simulink model "ArduCopter_MinnieTrajController"  (R2018b)
settings: Solver=FixedStepDiscrete  StartTime=0.0  StopTime=1000  FixedStep=cntrl.sample_time  RelTol=1e-4
undefined symbols (not defined in the file): cycle, DiscIntNeverNeededParam, fm_loiter, traj_empty
libraries: simulink x6, ndi_lib x5, axes_transformation_lib x4, angles_lib x3, ardupilot_custom_controller_lib x2, filters_lib x2, cntrl_atti_red_indi_lib x2, traj_lib x2, control_allocation_lib x1, dspsigops x1
(part 1 of 2)
settings Model: Creator=Yannic  LastModifiedBy=eike
settings SolverCC: ZeroCrossControl=DisableAll
settings DataIOCC: LimitDataPoints=on  SaveOutput=off  SaveTime=off  ReturnWorkspaceOutputs=on
settings OptimizationCC: DefaultParameterBehavior=Inlined  UseFloatMulNetSlope=on  DefaultUnderspecifiedDataType=single  InlineInvariantSignals=on  PassReuseOutputArgsAs=Individual arguments  ZeroExternalMemoryAtStartup=off  ZeroInternalMemoryAtStartup=off  NoFixptDivByZeroProtection=on  EfficientFloat2IntCast=on  LifeSpan=1  OptimizeBlockOrder=speed  DifferentSizesBufferReuse=on
settings DebuggingCC: ReadBeforeWriteMsg=DisableAll  WriteAfterWriteMsg=DisableAll  WriteAfterReadMsg=DisableAll  MultiTaskDSMMsg=none  ParameterTunabilityLossMsg=error  AllowSymbolicDim=off  LibraryContextMissingDiagnostic=none  SFUnexpectedBacktrackingDiag=warning  SFNoUnconditionalDefaultTransitionDiag=warning  SFExecutionAtInitializationDiag=none
settings HardwareCC: ProdBitPerPointer=32  ProdBitPerSizeT=32  ProdBitPerPtrDiffT=32  ProdLargestAtomicInteger=Long  ProdLargestAtomicFloat=Double  ProdWordSize=32  ProdHWDeviceType=ARM Compatible->ARM Cortex
settings ModelReferenceCC: UpdateModelReferenceTargets=IfOutOfDate  PropagateSignalLabelsOutOfModel=off
settings SFSimCC: SFSimEcho=off  SimUseLocalCustomCode=off  MATLABDynamicMemAlloc=off
settings RTWCC: SystemTargetFile=ert.tlc  GenCodeOnly=on  TemplateMakefile=ert_default_tmf  GenerateReport=on  RTWUseLocalCustomCode=off  IncludeHyperlinkInReport=on  LaunchReport=on  TargetLang=C++  GenerateTraceInfo=on  GenerateTraceReport=on  GenerateTraceReportSl=on  GenerateTraceReportSf=on  GenerateTraceReportEml=on
settings CodeAppCC: ForceParamTrailComments=on  IgnoreCustomStorageClasses=off  OperatorAnnotations=on  SimulinkDataObjDesc=on  SFDataObjDesc=on  CustomSymbolStrGlobalVar=rt$N$M  CustomSymbolStrType=$N$M  CustomSymbolStrFcn=$N$M$F  CustomSymbolStrMacro=$N$M  InsertBlockDesc=on
settings ERTTargetCC: TargetLangStandard=C++03 (ISO)  GenerateSampleERTMain=on  IncludeMdlTerminateFcn=off  CombineSignalStateStructs=on  SuppressErrorStatus=on  SupportAbsoluteTime=off  MultiInstanceERTCode=on  CodeInterfacePackaging=C++ class  SupportVariableSizeSignals=on  ERTHeaderFileRootName=MatlabController$E  ERTSourceFileRootName=MatlabController$E  ERTDataFileRootName=MatlabController_data  InlinedParameterPlacement=NonHierarchical  RootIOFormat=Structure reference  ERTCustomFileTemplate=example_file_process.tlc  ERTFilePackagingFormat=CompactWithDataFile
settings ConfigComp: CovMetricSettings=dw  CovHtmlReporting=on  CovSaveCumulativeToWorkspaceVar=on  CovSaveSingleToWorkspaceVar=on  CovExternalEMLEnable=off

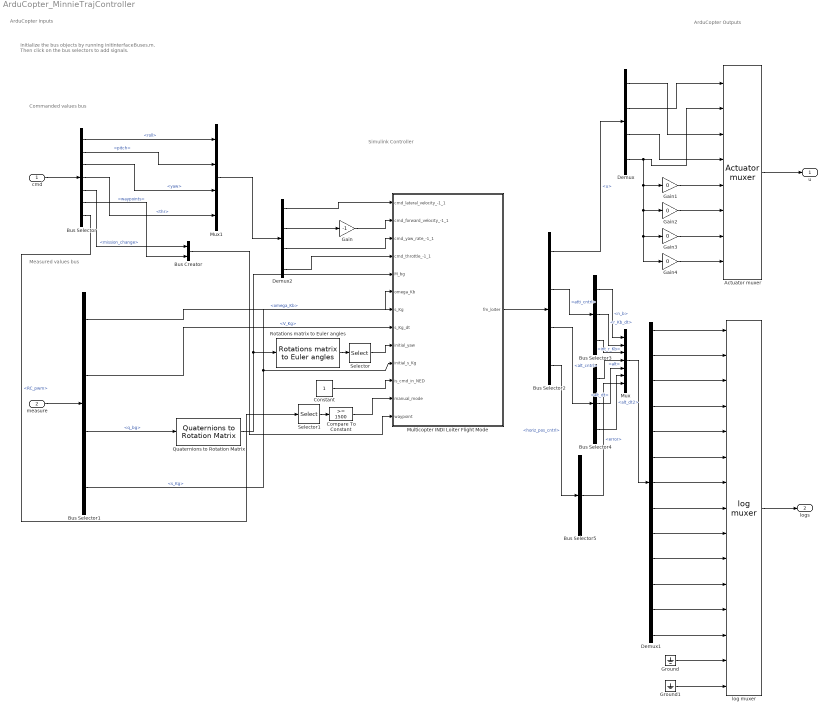
== system ArduCopter_MinnieTrajController ==
  note: Measured values bus
  note: Initialize the bus objects by running initInterfaceBuses.m.
      | Then click on the bus selectors to add signals.
  note: Commanded values bus
  note: ArduCopter Inputs
  note: ArduCopter Outputs
  note: Simulink Controller
  cmd : Inport  OutDataTypeStr=Bus: cmdBus
  measure : Inport  Port=2  OutDataTypeStr=Bus: measureBus
  Actuator muxer : ardupilot_custom_controller_lib/Actuator muxer
      settings: SourceProductName=LADAC
  Bus Creator : BusCreator  Inputs=2
  Bus Selector : BusSelector  OutputSignals=roll,pitch,yaw,thr,mission_change,waypoints,RC_pwm
  Bus Selector1 : BusSelector  OutputSignals=omega_Kb,V_Kg,q_bg,s_Kg
  Bus Selector2 : BusSelector  OutputSignals=fm_alt_hold.u,fm_alt_hold.atti_cntrl,fm_alt_hold.alt_cntrl,horiz_pos_cntrl
  Bus Selector3 : BusSelector  OutputSignals=error.n_b,error.r_Kb_dt,error.int_r_Kb
  Bus Selector4 : BusSelector  OutputSignals=error.alt,error.alt_dt,error.alt_dt2
  Bus Selector5 : BusSelector  OutputSignals=error
  Compare To Constant : simulink/Logic and Bit Operations/Compare To Constant  relop=>=  const=1500  OutDataTypeStr=boolean
  Constant : Constant
  Demux : Demux
  Demux1 : Demux  Outputs=13
  Demux2 : Demux
  Gain : Gain  Gain=-1
  Gain{1..4} (4 alike) : Gain  Gain=0
  Ground : Ground
  Ground1 : Ground
  Multicopter INDI Loiter Flight Mode : Subsystem  AncestorBlock=fm_copter_loiter_indi_lib/Multicopter INDI Loiter Flight Mode  mask{fm=fm_loiter}
      mask prompts: fm "Multicopter INDI loiter flight  struct"
      mask DialogControl DescGroupVar Prompt: Multicopter INDI Loiter Flight Mode
      mask DialogControl DescTextVar Prompt: Loiter flight mode using the reduced attitude controller with INDI.
      mask DialogControl Control2 Prompt: To intialize the parameters struct see multicopterFlightModeLoiter.
  Mux : Mux  Inputs=7
  Mux1 : Mux
  Quaternions to Rotation Matrix : axes_transformation_lib/Quaternions to Rotation Matrix  SystemSampleTime=-1
      settings: SourceProductName=LADAC
  Rotations matrix to Euler angles : axes_transformation_lib/Rotations matrix to Euler angles  SystemSampleTime=-1
      settings: SourceProductName=LADAC
  Selector : Selector  InputPortWidth=3  IndexOptions=Index vector (dialog)  Indices=3  OutputSizes=1
  Selector1 : Selector  InputPortWidth=16  IndexOptions=Index vector (dialog)  Indices=7  OutputSizes=1
  log muxer : ardupilot_custom_controller_lib/log muxer
      settings: SourceProductName=LADAC
  u : Outport  OutDataTypeStr=single
  logs : Outport  Port=2  OutDataTypeStr=single
  wires:
  cmd/1 -> Bus Selector/1
  measure/1 -> Bus Selector1/1
  Bus Selector/1 -> Mux1/1  "<roll>"
  Bus Selector/2 -> Mux1/2  "<pitch>"
  Bus Selector/3 -> Mux1/3  "<yaw>"
  Bus Selector/4 -> Mux1/4  "<thr>"
  Actuator muxer/1 -> u/1
  log muxer/1 -> logs/1
  Demux/4 -> Actuator muxer/2, Gain1/1, Gain4/1, Gain3/1, Gain2/1
  Gain1/1 -> Actuator muxer/5
  Demux/3 -> Actuator muxer/4
  Demux/2 -> Actuator muxer/1
  Demux1/1 -> log muxer/1
  Demux1/2 -> log muxer/2
  Demux1/3 -> log muxer/3
  Demux1/4 -> log muxer/4
  Demux1/5 -> log muxer/5
  Demux1/6 -> log muxer/6
  Demux1/7 -> log muxer/7
  Demux1/8 -> log muxer/8
  Demux1/9 -> log muxer/9
  Demux1/10 -> log muxer/10
  Demux1/11 -> log muxer/11
  Demux1/12 -> log muxer/12
  Demux1/13 -> log muxer/13
  Ground/1 -> log muxer/14
  Ground1/1 -> log muxer/15
  Gain/1 -> Multicopter INDI Loiter Flight Mode/2(cmd_forward_velocity_-1_1)
  Quaternions to Rotation Matrix/1 -> Multicopter INDI Loiter Flight Mode/5(M_bg), Rotations matrix to Euler angles/1
  Bus Selector1/2 -> Multicopter INDI Loiter Flight Mode/8(s_Kg_dt)  "<V_Kg>"
  Rotations matrix to Euler angles/1 -> Selector/1
  Mux1/1 -> Demux2/1
  Bus Selector1/1 -> Multicopter INDI Loiter Flight Mode/6(omega_Kb)  "<omega_Kb>"
  Demux2/2 -> Gain/1
  Demux2/3 -> Multicopter INDI Loiter Flight Mode/3(cmd_yaw_rate_-1_1)
  Bus Selector1/4 -> Multicopter INDI Loiter Flight Mode/10(initial_s_Kg), Multicopter INDI Loiter Flight Mode/7(s_Kg)  "<s_Kg>"
  Constant/1 -> Multicopter INDI Loiter Flight Mode/11(is_cmd_in_NED)
  Demux2/1 -> Multicopter INDI Loiter Flight Mode/1(cmd_lateral_velocity_-1_1)
  Bus Selector1/3 -> Quaternions to Rotation Matrix/1  "<q_bg>"
  Multicopter INDI Loiter Flight Mode/1(fm_loiter) -> Bus Selector2/1
  Bus Selector2/1 -> Demux/1  "<u>"
  Gain2/1 -> Actuator muxer/6
  Gain3/1 -> Actuator muxer/7
  Gain4/1 -> Actuator muxer/8
  Demux/1 -> Actuator muxer/3
  Bus Selector2/2 -> Bus Selector3/1  "<atti_cntrl>"
  Bus Selector2/3 -> Bus Selector4/1  "<alt_cntrl>"
  Bus Selector2/4 -> Bus Selector5/1  "<horiz_pos_cntrl>"
  Bus Selector5/1 -> Mux/7  "<error>"
  Bus Selector3/1 -> Mux/1  "<n_b>"
  Bus Selector3/3 -> Mux/3  "<int_r_Kb>"
  Bus Selector4/1 -> Mux/4  "<alt>"
  Bus Selector4/3 -> Mux/6  "<alt_dt2>"
  Mux/1 -> Demux1/1
  Bus Selector4/2 -> Mux/5  "<alt_dt>"
  Bus Selector3/2 -> Mux/2  "<r_Kb_dt>"
  Selector/1 -> Multicopter INDI Loiter Flight Mode/9(initial_yaw)
  Bus Selector/5 -> Bus Creator/1  "<mission_change>"
  Bus Selector/6 -> Bus Creator/2  "<waypoints>"
  Bus Selector/7 -> Selector1/1  "<RC_pwm>"
  Selector1/1 -> Compare To Constant/1
  Compare To Constant/1 -> Multicopter INDI Loiter Flight Mode/12(manual_mode)
  Bus Creator/1 -> Multicopter INDI Loiter Flight Mode/13(waypoint)
  Demux2/4 -> Multicopter INDI Loiter Flight Mode/4(cmd_throttle_-1_1)

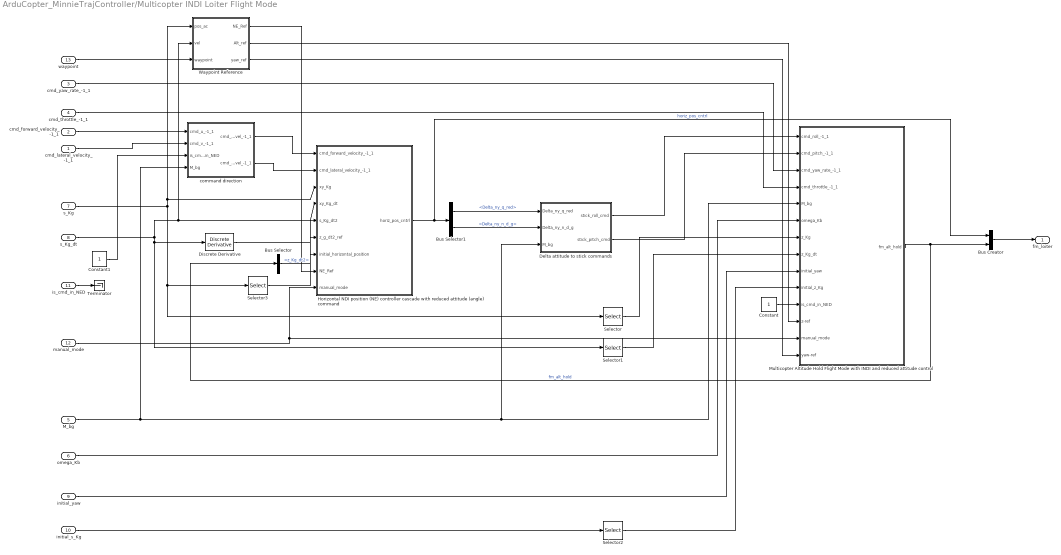
== system ArduCopter_MinnieTrajController/Multicopter INDI Loiter Flight Mode ==
  cmd_lateral_velocity_-1_1 : Inport  SampleTime=fm.sample_time
  cmd_forward_velocity_-1_1 : Inport  Port=2  SampleTime=fm.sample_time
  cmd_yaw_rate_-1_1 : Inport  Port=3  SampleTime=fm.sample_time
  cmd_throttle_-1_1 : Inport  Port=4  SampleTime=fm.sample_time
  M_bg : Inport  Port=5  SampleTime=fm.sample_time
  omega_Kb : Inport  Port=6  SampleTime=fm.sample_time
  s_Kg : Inport  Port=7  SampleTime=fm.sample_time
  s_Kg_dt : Inport  Port=8  SampleTime=fm.sample_time
  initial_yaw : Inport  Port=9  SampleTime=fm.sample_time
  initial_s_Kg : Inport  Port=10  SampleTime=fm.sample_time
  is_cmd_in_NED : Inport  Port=11  SampleTime=fm.sample_time
  manual_mode : Inport  Port=12
  waypoint : Inport  Port=13
  Bus Creator : BusCreator  Inputs=2
  Bus Selector : BusSelector  OutputSignals=alt_cntrl.reference.z_Kg_dt2
  Bus Selector1 : BusSelector  OutputSignals=pseudo_control.Delta_ny_q_red,pseudo_control.Delta_ny_n_d_g
  Constant : Constant
  Constant1 : Constant  OutDataTypeStr=Inherit: Inherit via back propagation
  Delta attitude to stick commands : Subsystem
  Discrete Derivative : simulink/Discrete/Discrete Derivative  gainval=1.0  ICPrevScaledInput=0.0  OutMin=[]  OutMax=[]  OutDataType=fixdt(1, 16)  OutScaling=2^-10  DoSatur=off
  Horizontal NDI position (NE) controller cascade with reduced attitude (angle) command : Subsystem  AncestorBlock=|  mask{horiz_pos_cntrl=fm.horiz_pos_cntrl, T=2./fm.fm_alt.cntrl.atti_cntrl.rm.lean.omega + fm.fm_alt.motor_time_constant + 2./fm.fm_alt.sens_filt.omega}
      | cntrl_horiz_pos_indi_lib/Horizontal NDI position (NE) controller cascade
      | with reduced attitude (angle) command
      mask prompts: horiz_pos_cntrl "horizontal position controller struct"; T "inner loop time constant"
      mask DialogControl DescGroupVar Prompt: Horizontal position controller cascade
      mask DialogControl DescTextVar Prompt: The commanded velocity is filtered and the control error is converted into desired accerlations in x_g and y_g direction. The commanded accelerations are converted into commanded to reduced attitude angles.
      mask DialogControl Control2 Prompt: To initialize a horizontal position controller parameters struct see cntrlHorizPosIndiLoadParams
  Multicopter Altitude Hold Flight Mode with INDI and reduced attitude control : Subsystem  AncestorBlock=fm_copter_alt_hold_indi_lib/Multicopter Altitude Hold Flight Mode with INDI and reduced attitude control  mask{fm=fm.fm_alt}
      mask prompts: fm "Multicopter Altitude Hold Flight Mode (INDI) struct"
      mask DialogControl DescGroupVar Prompt: Multicopter Attitude Flight Mode with INDI and reduced attitude control
      mask DialogControl DescTextVar Prompt: Controller is basically implemented according to [1]
      mask DialogControl Control2 Prompt: [1] Sun, S., Baert, M., Van Schijndel, B. S., & De Visser, C. (2020, May). Upset Recovery Control for Quadrotors Subjected to a Complete Rotor Failure from Large Initial Disturbances. In 2020 IEEE International Conference on Robotics and Automation (ICRA) (pp. 4273-4279). IEEE.
      mask DialogControl Control3 Prompt: To initialize an altitude hold flight mode struct see fmCopterAltHoldIndiLoadParams
  Selector : Selector  InputPortWidth=3  IndexOptions=Index vector (dialog)  Indices=3  OutputSizes=1
  Selector1 : Selector  InputPortWidth=3  IndexOptions=Index vector (dialog)  Indices=3  OutputSizes=1
  Selector2 : Selector  InputPortWidth=3  IndexOptions=Index vector (dialog)  Indices=3  OutputSizes=1
  Selector3 : Selector  InputPortWidth=3  IndexOptions=Index vector (dialog)  Indices=[1,2]  OutputSizes=1
  Terminator : Terminator
  Waypoint Reference : Subsystem
  command direction : Subsystem
  fm_loiter : Outport  OutDataTypeStr=single  SampleTime=fm.sample_time
  wires:
  is_cmd_in_NED/1 -> Terminator/1
  command direction/2(cmd_east_vel_-1_1) -> Horizontal NDI position (NE) controller cascade with reduced attitude (angle) command/2(cmd_lateral_velocity_-1_1)
  command direction/1(cmd_north_vel_-1_1) -> Horizontal NDI position (NE) controller cascade with reduced attitude (angle) command/1(cmd_forward_velocity_-1_1)
  Bus Creator/1 -> fm_loiter/1
  Bus Selector1/1 -> Delta attitude to stick commands/1(Delta_ny_q_red)  "<Delta_ny_q_red>"
  Selector2/1 -> Multicopter Altitude Hold Flight Mode with INDI and reduced attitude control/10(initial_z_Kg)
  Constant1/1 -> command direction/3(is_cmd_in_NED)
  Delta attitude to stick commands/1(stick_roll_cmd) -> Multicopter Altitude Hold Flight Mode with INDI and reduced attitude control/1(cmd_roll_-1_1)
  Selector/1 -> Multicopter Altitude Hold Flight Mode with INDI and reduced attitude control/7(z_Kg)
  cmd_lateral_velocity_-1_1/1 -> command direction/2(cmd_v_-1_1)
  Bus Selector/1 -> Horizontal NDI position (NE) controller cascade with reduced attitude (angle) command/6(z_g_dt2_ref)  "<z_Kg_dt2>"
  cmd_throttle_-1_1/1 -> Multicopter Altitude Hold Flight Mode with INDI and reduced attitude control/4(cmd_throttle_-1_1)
  initial_yaw/1 -> Multicopter Altitude Hold Flight Mode with INDI and reduced attitude control/9(initial_yaw)
  Delta attitude to stick commands/2(stick_pitch_cmd) -> Multicopter Altitude Hold Flight Mode with INDI and reduced attitude control/2(cmd_pitch_-1_1)
  s_Kg/1 -> Selector/1, Selector3/1, Waypoint Reference/1(pos_ac), Horizontal NDI position (NE) controller cascade with reduced attitude (angle) command/3(xy_Kg)
  Selector1/1 -> Multicopter Altitude Hold Flight Mode with INDI and reduced attitude control/8(z_Kg_dt)
  Multicopter Altitude Hold Flight Mode with INDI and reduced attitude control/1(fm_alt_hold) -> Bus Selector/1, Bus Creator/2  "fm_alt_hold"
  M_bg/1 -> command direction/4(M_bg), Multicopter Altitude Hold Flight Mode with INDI and reduced attitude control/5(M_bg), Delta attitude to stick commands/3(M_bg)
  Bus Selector1/2 -> Delta attitude to stick commands/2(Delta_ny_n_d_g)  "<Delta_ny_n_d_g>"
  Horizontal NDI position (NE) controller cascade with reduced attitude (angle) command/1(horiz_pos_cntrl) -> Bus Selector1/1, Bus Creator/1  "horiz_pos_cntrl"
  omega_Kb/1 -> Multicopter Altitude Hold Flight Mode with INDI and reduced attitude control/6(omega_Kb)
  initial_s_Kg/1 -> Selector2/1
  Selector3/1 -> Horizontal NDI position (NE) controller cascade with reduced attitude (angle) command/7(initial_horizontal_position)
  Constant/1 -> Multicopter Altitude Hold Flight Mode with INDI and reduced attitude control/11(is_cmd_in_NED)
  cmd_yaw_rate_-1_1/1 -> Multicopter Altitude Hold Flight Mode with INDI and reduced attitude control/3(cmd_yaw_rate_-1_1)
  Discrete Derivative/1 -> Horizontal NDI position (NE) controller cascade with reduced attitude (angle) command/5(s_Kg_dt2)
  s_Kg_dt/1 -> Selector1/1, Discrete Derivative/1, Horizontal NDI position (NE) controller cascade with reduced attitude (angle) command/4(xy_Kg_dt), Waypoint Reference/2(vel)
  cmd_forward_velocity_-1_1/1 -> command direction/1(cmd_u_-1_1)
  Waypoint Reference/1(NE_Ref) -> Horizontal NDI position (NE) controller cascade with reduced attitude (angle) command/8(NE_Ref)
  manual_mode/1 -> Horizontal NDI position (NE) controller cascade with reduced attitude (angle) command/9(manual_mode), Multicopter Altitude Hold Flight Mode with INDI and reduced attitude control/13(manual_mode)
  Waypoint Reference/2(Alt_ref) -> Multicopter Altitude Hold Flight Mode with INDI and reduced attitude control/12(z-ref)
  Waypoint Reference/3(yaw_ref) -> Multicopter Altitude Hold Flight Mode with INDI and reduced attitude control/14(yaw-ref)
  waypoint/1 -> Waypoint Reference/3(waypoint)

== system ArduCopter_MinnieTrajController/Multicopter INDI Loiter Flight Mode/Delta attitude to stick commands ==
  Delta_ny_q_red : Inport
  Delta_ny_n_d_g : Inport  Port=2
  M_bg : Inport  Port=3
  Gain : Gain  Gain=1/fm.fm_alt.cntrl.atti_cntrl.rm.lean.max
  MATLAB Function1 : MATLAB Function  TreatAsAtomicUnit=on
  Saturation : Saturate  UpperLimit=fm.fm_alt.cntrl.atti_cntrl.rm.lean.max  LowerLimit=0
  conversion to total attitude command : Subsystem
  stick_roll_cmd : Outport
  stick_pitch_cmd : Outport  Port=2
  wires:
  Gain/1 -> MATLAB Function1/1(lean_angle_0_1)
  M_bg/1 -> conversion to total attitude command/3(M_bg)
  Delta_ny_q_red/1 -> conversion to total attitude command/1(Delta_q)
  Delta_ny_n_d_g/1 -> conversion to total attitude command/2(Delta_n_g)
  MATLAB Function1/2(stick_pitch_cmd) -> stick_pitch_cmd/1
  MATLAB Function1/1(stick_roll_cmd) -> stick_roll_cmd/1
  conversion to total attitude command/1(lean_angle) -> Saturation/1
  conversion to total attitude command/2(lean_direction_angle) -> MATLAB Function1/2(lean_direction_angle)
  Saturation/1 -> Gain/1

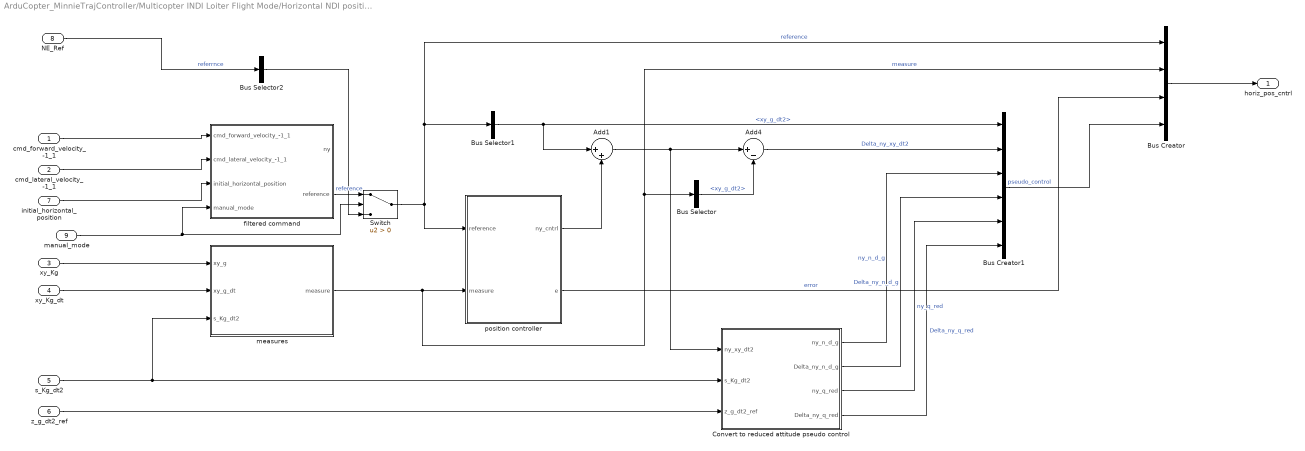
== system ArduCopter_MinnieTrajController/Multicopter INDI Loiter Flight Mode/Horizontal NDI position (NE) controller cascade with reduced attitude (angle) command ==
  cmd_forward_velocity_-1_1 : Inport
  cmd_lateral_velocity_-1_1 : Inport  Port=2
  xy_Kg : Inport  Port=3
  xy_Kg_dt : Inport  Port=4
  s_Kg_dt2 : Inport  Port=5
  z_g_dt2_ref : Inport  Port=6
  initial_horizontal_position : Inport  Port=7
  NE_Ref : Inport  Port=8
  manual_mode : Inport  Port=9
  Add1 : Sum  Inputs=|++
  Add4 : Sum  Inputs=|+-
  Bus Creator : BusCreator  Inputs=4
  Bus Creator1 : BusCreator  Inputs=6
  Bus Selector : BusSelector  OutputSignals=xy_g_dt2
  Bus Selector1 : BusSelector  OutputSignals=xy_g_dt2
  Bus Selector2 : BusSelector  OutputSignals=xy_g,xy_g_dt,xy_g_dt2  OutputAsBus=on
  Convert to reduced attitude pseudo control : Subsystem
  Switch : Switch  Criteria=u2 > Threshold
  filtered command : Subsystem
  measures : Subsystem
  position controller : Subsystem
  horiz_pos_cntrl : Outport
  wires:
  Convert to reduced attitude pseudo control/4(Delta_ny_q_red) -> Bus Creator1/6  "Delta_ny_q_red"
  Convert to reduced attitude pseudo control/3(ny_q_red) -> Bus Creator1/5  "ny_q_red"
  Convert to reduced attitude pseudo control/2(Delta_ny_n_d_g) -> Bus Creator1/4  "Delta_ny_n_d_g"
  Convert to reduced attitude pseudo control/1(ny_n_d_g) -> Bus Creator1/3  "ny_n_d_g"
  z_g_dt2_ref/1 -> Convert to reduced attitude pseudo control/3(z_g_dt2_ref)
  Bus Creator/1 -> horiz_pos_cntrl/1
  Bus Creator1/1 -> Bus Creator/4  "pseudo_control"
  Bus Selector/1 -> Add4/2  "<xy_g_dt2>"
  Add4/1 -> Bus Creator1/2  "Delta_ny_xy_dt2"
  measures/1(measure) -> position controller/2(measure), Bus Selector/1, Bus Creator/2  "measure"
  cmd_lateral_velocity_-1_1/1 -> filtered command/2(cmd_lateral_velocity_-1_1)
  xy_Kg_dt/1 -> measures/2(xy_g_dt)
  xy_Kg/1 -> measures/1(xy_g)
  position controller/2(e) -> Bus Creator/3  "error"
  s_Kg_dt2/1 -> Convert to reduced attitude pseudo control/2(s_Kg_dt2), measures/3(s_Kg_dt2)
  Add1/1 -> Add4/1, Convert to reduced attitude pseudo control/1(ny_xy_dt2)
  position controller/1(ny_cntrl) -> Add1/2
  initial_horizontal_position/1 -> filtered command/3(initial_horizontal_position)
  Switch/1 -> Bus Creator/1, Bus Selector1/1, position controller/1(reference)  "reference"
  cmd_forward_velocity_-1_1/1 -> filtered command/1(cmd_forward_velocity_-1_1)
  Bus Selector1/1 -> Add1/1, Bus Creator1/1  "<xy_g_dt2>"
  NE_Ref/1 -> Bus Selector2/1  "referrnce"
  Bus Selector2/1 -> Switch/3
  filtered command/2(reference) -> Switch/1  "reference"
  manual_mode/1 -> filtered command/4(manual_mode), Switch/2

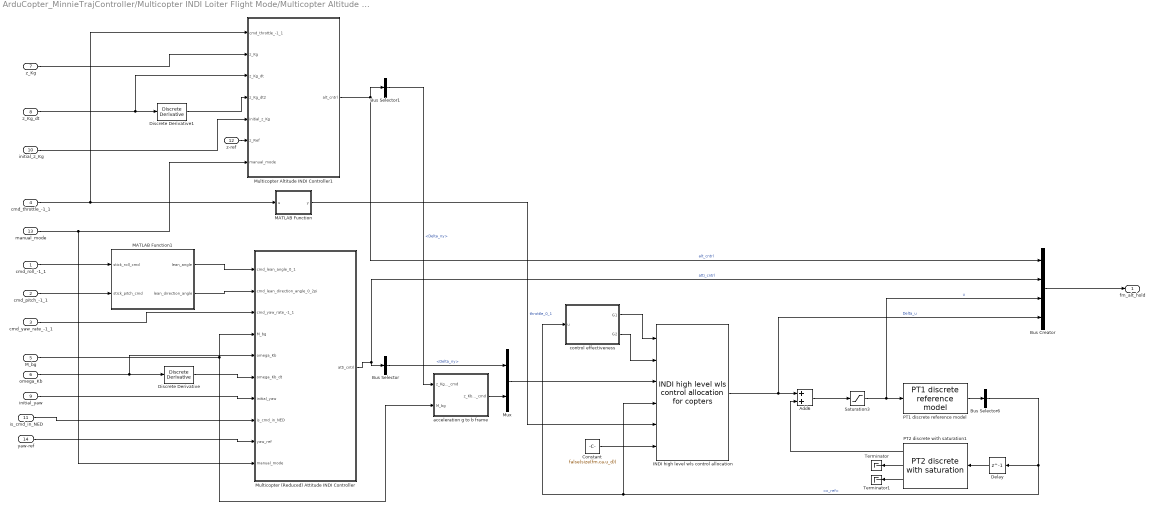
== system ArduCopter_MinnieTrajController/Multicopter INDI Loiter Flight Mode/Multicopter Altitude Hold Flight Mode with INDI and reduced attitude control ==
  cmd_roll_-1_1 : Inport  SampleTime=fm.sample_time
  cmd_pitch_-1_1 : Inport  Port=2  SampleTime=fm.sample_time
  cmd_yaw_rate_-1_1 : Inport  Port=3  SampleTime=fm.sample_time
  cmd_throttle_-1_1 : Inport  Port=4  SampleTime=fm.sample_time
  M_bg : Inport  Port=5  SampleTime=fm.sample_time
  omega_Kb : Inport  Port=6  SampleTime=fm.sample_time
  z_Kg : Inport  Port=7  SampleTime=fm.sample_time
  z_Kg_dt : Inport  Port=8  SampleTime=fm.sample_time
  initial_yaw : Inport  Port=9  SampleTime=fm.sample_time
  initial_z_Kg : Inport  Port=10  SampleTime=fm.sample_time
  is_cmd_in_NED : Inport  Port=11  SampleTime=fm.sample_time
  z-ref : Inport  Port=12
  manual_mode : Inport  Port=13
  yaw-ref : Inport  Port=14
  Add6 : Sum
  Bus Creator : BusCreator  Inputs=4
  Bus Selector : BusSelector  OutputSignals=pseudo_control.Delta_ny
  Bus Selector1 : BusSelector  OutputSignals=pseudo_control.Delta_ny
  Bus Selector6 : BusSelector  OutputSignals=x_ref
  Constant : Constant  Value=false(size(fm.ca.u_d))
  Delay : Delay  DelayLength=1
  Discrete Derivative : simulink/Discrete/Discrete Derivative  gainval=1.0  ICPrevScaledInput=0.0  OutMin=[]  OutMax=[]  OutDataType=fixdt(1, 16)  OutScaling=2^-10  DoSatur=off
  Discrete Derivative1 : simulink/Discrete/Discrete Derivative  gainval=1.0  ICPrevScaledInput=0.0  OutMin=[]  OutMax=[]  OutDataType=fixdt(1, 16)  OutScaling=2^-10  DoSatur=off
  INDI high level wls control allocation : control_allocation_lib/INDI high level wls control allocation for copters  ca=fm.ca
  MATLAB Function : MATLAB Function  TreatAsAtomicUnit=on
  MATLAB Function1 : MATLAB Function  TreatAsAtomicUnit=on
  Multicopter (Reduced) Attitude INDI Controller : Subsystem  AncestorBlock=cntrl_atti_red_indi_lib/Multicopter (Reduced) Attitude INDI Controller  mask{atti_cntrl=fm.cntrl.atti_cntrl, T=fm.motor_time_constant + 2./fm.sens_filt.omega}
      mask prompts: atti_cntrl "reduced attitude control struct"; T "inner loop time constant"
      mask Help: https://www.mathworks.com
      mask DialogControl DescGroupVar Prompt: INDI Reduced Attitude Controller
      mask DialogControl DescTextVar Prompt: To initialize the reduced attitude control struct see cntrlAttiRedIndiLoadParams
  Multicopter Altitude INDI Controller1 : Subsystem  AncestorBlock=cntrl_alt_indi/Multicopter Altitude INDI Controller  mask{alt_cntrl=fm.cntrl}
      mask prompts: alt_cntrl "reduced attitude control struct"
      mask DialogControl DescGroupVar Prompt: INDI Reduced Attitude Controller
      mask DialogControl DescTextVar Prompt: To initialize the reduced attitude control struct see cntrlAttiRedIndiLoadParams.
  Mux : Mux  Inputs=2
  PT1 discrete reference model : ndi_lib/PT1 discrete reference model  T=fm.motor_time_constant  x_max=inf  x_min=-inf  x_dt_max=inf  x_dt_min=-inf  x_init=0
      settings: SourceProductName=LADAC
  PT2 discrete with saturation1 : filters_lib/PT2 discrete with saturation  omega=fm.sens_filt.omega  d=fm.sens_filt.D  x_dt2_max=inf  x_dt2_min=-inf  x_dt_max=inf  x_dt_min=-inf  x_max=inf  x_min=-inf  x_init=0  x_dt_init=0
      settings: SourceProductName=LADAC
  Saturation3 : Saturate  UpperLimit=fm.ca.u_max  LowerLimit=fm.ca.u_min
  Terminator : Terminator
  Terminator1 : Terminator
  acceleration g to b frame : Subsystem
  control effectiveness : Subsystem
  fm_alt_hold : Outport  OutDataTypeStr=single  SampleTime=fm.sample_time
  wires:
  PT2 discrete with saturation1/1 -> Add6/2
  acceleration g to b frame/1(z_Kb_dt2_cmd) -> Mux/2
  M_bg/1 -> Multicopter (Reduced) Attitude INDI Controller/4(M_bg), acceleration g to b frame/2(M_bg)
  INDI high level wls control allocation/1 -> Add6/1, Bus Creator/4  "Delta_u"
  Mux/1 -> INDI high level wls control allocation/3
  cmd_pitch_-1_1/1 -> MATLAB Function1/2(stick_pitch_cmd)
  cmd_roll_-1_1/1 -> MATLAB Function1/1(stick_roll_cmd)
  Bus Creator/1 -> fm_alt_hold/1
  initial_z_Kg/1 -> Multicopter Altitude INDI Controller1/5(initial_z_Kg)
  Discrete Derivative1/1 -> Multicopter Altitude INDI Controller1/4(z_Kg_dt2)
  z_Kg_dt/1 -> Multicopter Altitude INDI Controller1/3(z_Kg_dt), Discrete Derivative1/1
  z_Kg/1 -> Multicopter Altitude INDI Controller1/2(z_Kg)
  PT2 discrete with saturation1/3 -> Terminator1/1
  PT2 discrete with saturation1/2 -> Terminator/1
  omega_Kb/1 -> Multicopter (Reduced) Attitude INDI Controller/5(omega_Kb), Discrete Derivative/1
  Discrete Derivative/1 -> Multicopter (Reduced) Attitude INDI Controller/6(omega_Kb_dt)
  Bus Selector/1 -> Mux/1  "<Delta_ny>"
  MATLAB Function1/1(lean_angle) -> Multicopter (Reduced) Attitude INDI Controller/1(cmd_lean_angle_0_1)
  initial_yaw/1 -> Multicopter (Reduced) Attitude INDI Controller/7(initial_yaw)
  Multicopter (Reduced) Attitude INDI Controller/1(atti_cntrl) -> Bus Selector/1, Bus Creator/2  "atti_cntrl"
  Bus Selector6/1 -> Delay/1, control effectiveness/1(u), INDI high level wls control allocation/4  "<x_ref>"
  control effectiveness/2(G2) -> INDI high level wls control allocation/2
  Add6/1 -> Saturation3/1
  cmd_throttle_-1_1/1 -> Multicopter Altitude INDI Controller1/1(cmd_throttle_-1_1), MATLAB Function/1(u)
  MATLAB Function/1(y) -> INDI high level wls control allocation/5  "throttle_0_1"
  Bus Selector1/1 -> acceleration g to b frame/1(z_Kg_dt2_cmd)  "<Delta_ny>"
  MATLAB Function1/2(lean_direction_angle) -> Multicopter (Reduced) Attitude INDI Controller/2(cmd_lean_direction_angle_0_2pi)
  Delay/1 -> PT2 discrete with saturation1/1
  Constant/1 -> INDI high level wls control allocation/6
  PT1 discrete reference model/1 -> Bus Selector6/1
  Saturation3/1 -> PT1 discrete reference model/1, Bus Creator/3  "u"
  cmd_yaw_rate_-1_1/1 -> Multicopter (Reduced) Attitude INDI Controller/3(cmd_yaw_rate_-1_1)
  Multicopter Altitude INDI Controller1/1(alt_cntrl) -> Bus Selector1/1, Bus Creator/1  "alt_cntrl"
  control effectiveness/1(G1) -> INDI high level wls control allocation/1
  is_cmd_in_NED/1 -> Multicopter (Reduced) Attitude INDI Controller/8(is_cmd_in_NED)
  z-ref/1 -> Multicopter Altitude INDI Controller1/6(z_Ref)
  manual_mode/1 -> Multicopter (Reduced) Attitude INDI Controller/10(manual_mode), Multicopter Altitude INDI Controller1/7(manual_mode)
  yaw-ref/1 -> Multicopter (Reduced) Attitude INDI Controller/9("yaw_ref ")

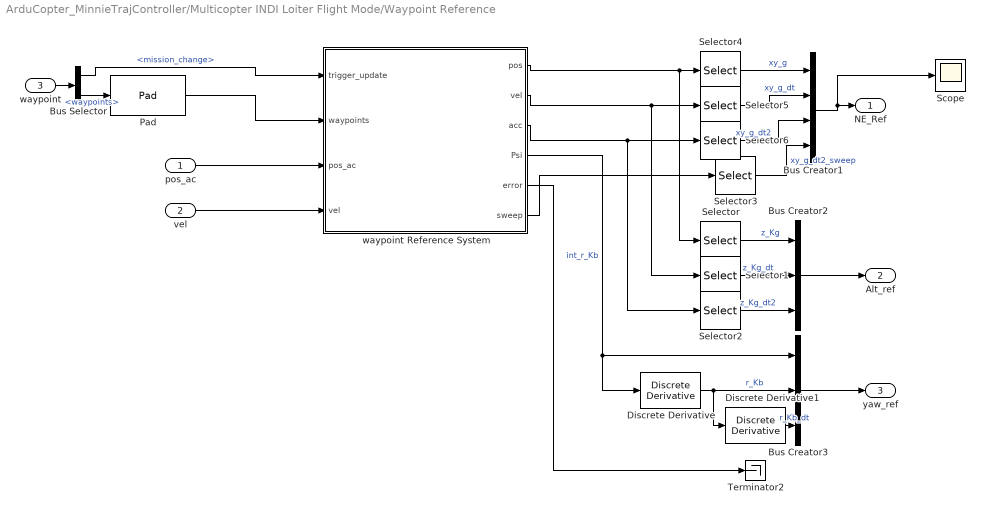
== system ArduCopter_MinnieTrajController/Multicopter INDI Loiter Flight Mode/Waypoint Reference ==
  pos_ac : Inport
  vel : Inport  Port=2
  waypoint : Inport  Port=3
  Bus Creator1 : BusCreator  Inputs=4
  Bus Creator2 : BusCreator  Inputs=3
  Bus Creator3 : BusCreator  Inputs=3
  Bus Selector : BusSelector  OutputSignals=mission_change,waypoints
  Discrete Derivative : simulink/Discrete/Discrete Derivative  gainval=1  ICPrevScaledInput=0.0  OutMin=[]  OutMax=[]  OutDataType=fixdt(1, 16)  OutScaling=2^-10  DoSatur=off
  Discrete Derivative1 : simulink/Discrete/Discrete Derivative  gainval=1  ICPrevScaledInput=0.0  OutMin=[]  OutMax=[]  OutDataType=fixdt(1, 16)  OutScaling=2^-10  DoSatur=off
  Pad : dspsigops/Pad  padAlong=Columns and rows  dimsToPad=1  valSrc=Specify via dialog  padVal=0  spec=Output size  padNumOutRowsSpecMethod=User-specified  numOutRows=3  padNumOutColsSpecMethod=User-specified  numOutCols=traj_size  isVarDimsMode=off  padBeginning=0  padEnd=0  outSizeMode=User-specified  outSize=1  padSigAt=End  trunc_flag=None  roundingMode=Floor  overflowMode=off  truncOrWrapMode=Truncate  wrap_flag=None
      settings: SourceProductName=DSP System Toolbox  SourceProductBaseCode=DS
  Scope : Scope
  Selector : Selector  InputPortWidth=3  IndexOptions=Index vector (dialog)  Indices=3  OutputSizes=1
  Selector1 : Selector  InputPortWidth=3  IndexOptions=Index vector (dialog)  Indices=3  OutputSizes=1
  Selector2 : Selector  InputPortWidth=3  IndexOptions=Index vector (dialog)  Indices=3  OutputSizes=1
  Selector{3..6} (4 alike) : Selector  InputPortWidth=3  IndexOptions=Index vector (dialog)  Indices=[1 2]  OutputSizes=1
  Terminator2 : Terminator
  waypoint Reference System : Subsystem
  NE_Ref : Outport
  Alt_ref : Outport  Port=2
  yaw_ref : Outport  Port=3
  wires:
  waypoint Reference System/2(vel) -> Selector1/1, Selector5/1
  Selector6/1 -> Bus Creator1/3  "xy_g_dt2"
  Bus Creator1/1 -> Scope/1, NE_Ref/1
  waypoint Reference System/1(pos) -> Selector/1, Selector4/1
  Selector4/1 -> Bus Creator1/1  "xy_g"
  waypoint Reference System/3(acc) -> Selector2/1, Selector6/1
  Bus Selector/1 -> waypoint Reference System/1(trigger_update)  "<mission_change>"
  Selector5/1 -> Bus Creator1/2  "xy_g_dt"
  Pad/1 -> waypoint Reference System/2(waypoints)
  waypoint Reference System/5(error) -> Terminator2/1
  waypoint Reference System/4(Psi) -> Discrete Derivative/1, Bus Creator3/1  "int_r_Kb"
  Selector/1 -> Bus Creator2/1  "z_Kg"
  Selector1/1 -> Bus Creator2/2  "z_Kg_dt"
  Selector2/1 -> Bus Creator2/3  "z_Kg_dt2"
  Bus Creator2/1 -> Alt_ref/1
  pos_ac/1 -> waypoint Reference System/3(pos_ac)
  Bus Creator3/1 -> yaw_ref/1
  Discrete Derivative/1 -> Discrete Derivative1/1, Bus Creator3/2  "r_Kb"
  Discrete Derivative1/1 -> Bus Creator3/3  "r_Kb_dt"
  vel/1 -> waypoint Reference System/4("vel ")
  waypoint Reference System/6("sweep ") -> Selector3/1
  Selector3/1 -> Bus Creator1/4  "xy_g_dt2_sweep"
  waypoint/1 -> Bus Selector/1
  Bus Selector/2 -> Pad/1  "<waypoints>"

== system ArduCopter_MinnieTrajController/Multicopter INDI Loiter Flight Mode/command direction ==
  cmd_u_-1_1 : Inport
  cmd_v_-1_1 : Inport  Port=2
  is_cmd_in_NED : Inport  Port=3
  M_bg : Inport  Port=4
  MATLAB Function : MATLAB Function  TreatAsAtomicUnit=on
  cmd_north_vel_-1_1 : Outport
  cmd_east_vel_-1_1 : Outport  Port=2
  wires:
  M_bg/1 -> MATLAB Function/4(M_bg)
  MATLAB Function/2(cmd_v_E) -> cmd_east_vel_-1_1/1
  MATLAB Function/1(cmd_u_N) -> cmd_north_vel_-1_1/1
  is_cmd_in_NED/1 -> MATLAB Function/3(is_NED)
  cmd_v_-1_1/1 -> MATLAB Function/2(cmd_v)
  cmd_u_-1_1/1 -> MATLAB Function/1(cmd_u)

== system ArduCopter_MinnieTrajController/Multicopter INDI Loiter Flight Mode/Delta attitude to stick commands/conversion to total attitude command ==
  Delta_q : Inport
  Delta_n_g : Inport  Port=2
  M_bg : Inport  Port=3
  Add : Sum
  DCM to quaternions : axes_transformation_lib/DCM to quaternions  SystemSampleTime=-1
      settings: SourceProductName=LADAC
  MATLAB Function : MATLAB Function  TreatAsAtomicUnit=on
  MATLAB Function1 : MATLAB Function  TreatAsAtomicUnit=on
  MATLAB Function4 : MATLAB Function  TreatAsAtomicUnit=on
  Scope : Scope  NumInputPorts=4
  quaternion to lean angles : Subsystem
  total reduced attitude command (quaternion) : MATLAB Function  TreatAsAtomicUnit=on
  lean_angle : Outport
  lean_direction_angle : Outport  Port=2
  wires:
  DCM to quaternions/1 -> total reduced attitude command (quaternion)/2(q_m)
  M_bg/1 -> MATLAB Function1/1(M_bg), DCM to quaternions/1
  quaternion to lean angles/1(phi) -> Scope/1
  total reduced attitude command (quaternion)/1(q_cmd) -> quaternion to lean angles/1(q_bg)
  Add/1 -> MATLAB Function/1(u)
  Delta_q/1 -> total reduced attitude command (quaternion)/1(q_e)
  MATLAB Function4/1(phi) -> lean_angle/1, Scope/3
  quaternion to lean angles/2(delta) -> Scope/2
  MATLAB Function4/2(delta) -> Scope/4, lean_direction_angle/1
  Delta_n_g/1 -> Add/1
  MATLAB Function1/1(n_g) -> Add/2
  MATLAB Function/1(y) -> MATLAB Function4/1(n_g)

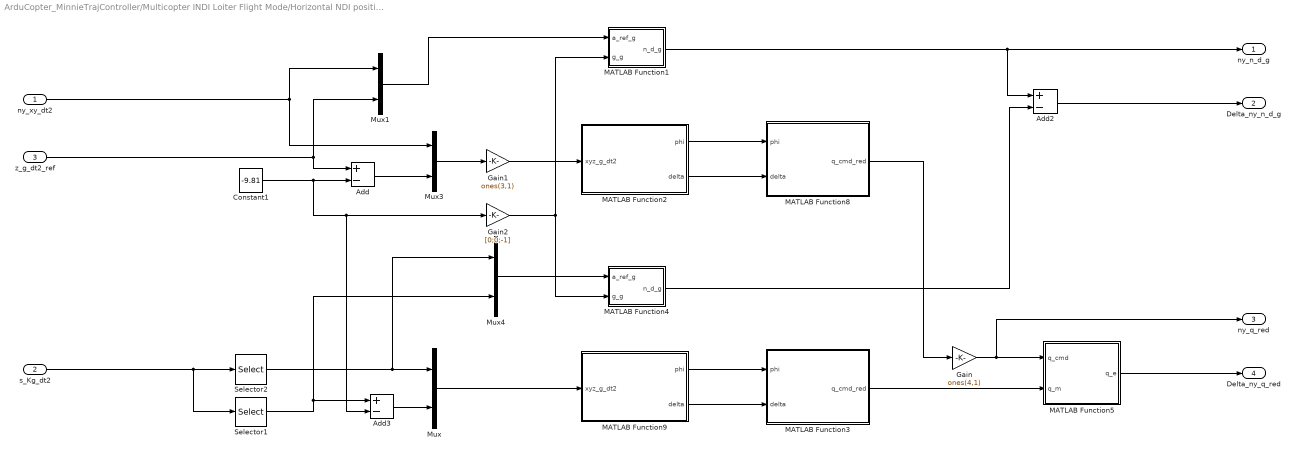
== system ArduCopter_MinnieTrajController/Multicopter INDI Loiter Flight Mode/Horizontal NDI position (NE) controller cascade with reduced attitude (angle) command/Convert to reduced attitude pseudo control ==
  ny_xy_dt2 : Inport
  s_Kg_dt2 : Inport  Port=2
  z_g_dt2_ref : Inport  Port=3
  Add : Sum  Inputs=+-
  Add2 : Sum  Inputs=+-
  Add3 : Sum  Inputs=+-
  Constant1 : Constant  Value=-9.81  OutDataTypeStr=single
  Gain : Gain  Gain=ones(4,1)
  Gain1 : Gain  Gain=ones(3,1)
  Gain2 : Gain  Gain=[0;0;-1]
  MATLAB Function1 : MATLAB Function  TreatAsAtomicUnit=on
  MATLAB Function2 : MATLAB Function  TreatAsAtomicUnit=on
  MATLAB Function3 : MATLAB Function  TreatAsAtomicUnit=on
  MATLAB Function4 : MATLAB Function  TreatAsAtomicUnit=on
  MATLAB Function5 : MATLAB Function  TreatAsAtomicUnit=on
  MATLAB Function8 : MATLAB Function  TreatAsAtomicUnit=on
  MATLAB Function9 : MATLAB Function  TreatAsAtomicUnit=on
  Mux{,1,3..4} (4 alike) : Mux  Inputs=2
  Selector1 : Selector  InputPortWidth=3  IndexOptions=Index vector (dialog)  Indices=3  OutputSizes=1
  Selector2 : Selector  InputPortWidth=3  IndexOptions=Index vector (dialog)  Indices=[1,2]  OutputSizes=1
  ny_n_d_g : Outport
  Delta_ny_n_d_g : Outport  Port=2
  ny_q_red : Outport  Port=3
  Delta_ny_q_red : Outport  Port=4
  wires:
  MATLAB Function2/1(phi) -> MATLAB Function8/1(phi)
  MATLAB Function8/1(q_cmd_red) -> Gain/1
  Gain/1 -> MATLAB Function5/1(q_cmd), ny_q_red/1
  MATLAB Function1/1(n_d_g) -> Add2/1, ny_n_d_g/1
  Constant1/1 -> Add3/2, Gain2/1, Add/2
  Mux3/1 -> Gain1/1
  ny_xy_dt2/1 -> Mux1/1, Mux3/1
  Mux1/1 -> MATLAB Function1/1(a_ref_g)
  MATLAB Function5/1(q_e) -> Delta_ny_q_red/1
  MATLAB Function9/1(phi) -> MATLAB Function3/1(phi)
  Gain2/1 -> MATLAB Function4/2(g_g), MATLAB Function1/2(g_g)
  Mux4/1 -> MATLAB Function4/1(a_ref_g)
  Add2/1 -> Delta_ny_n_d_g/1
  z_g_dt2_ref/1 -> Mux1/2, Add/1
  Gain1/1 -> MATLAB Function2/1(xyz_g_dt2)
  Add/1 -> Mux3/2
  MATLAB Function9/2(delta) -> MATLAB Function3/2(delta)
  s_Kg_dt2/1 -> Selector2/1, Selector1/1
  Add3/1 -> Mux/2
  Selector2/1 -> Mux4/1, Mux/1
  MATLAB Function4/1(n_d_g) -> Add2/2
  Selector1/1 -> Add3/1, Mux4/2
  MATLAB Function3/1(q_cmd_red) -> MATLAB Function5/2(q_m)
  MATLAB Function2/2(delta) -> MATLAB Function8/2(delta)
  Mux/1 -> MATLAB Function9/1(xyz_g_dt2)

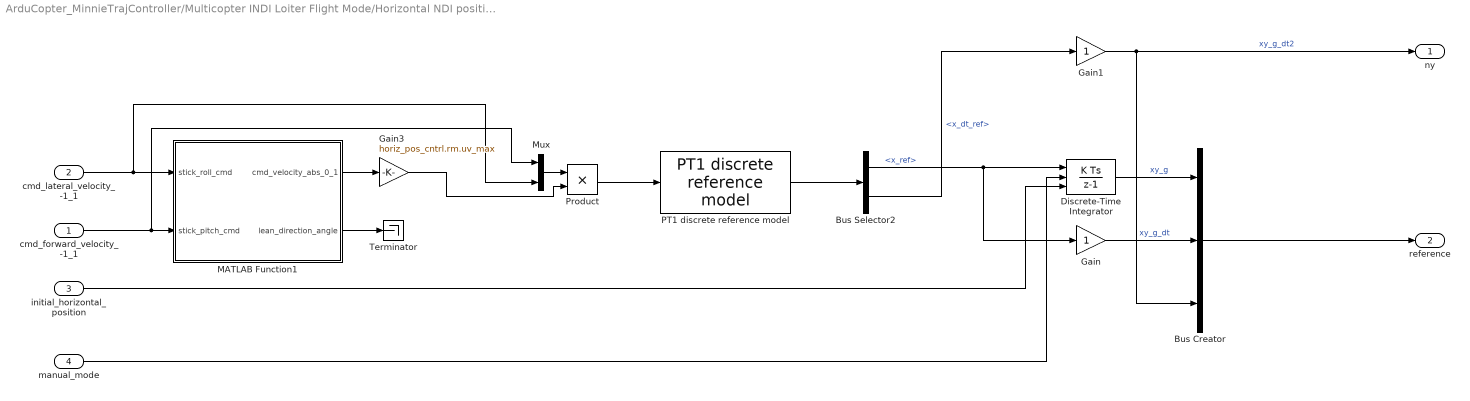
== system ArduCopter_MinnieTrajController/Multicopter INDI Loiter Flight Mode/Horizontal NDI position (NE) controller cascade with reduced attitude (angle) command/filtered command ==
  cmd_forward_velocity_-1_1 : Inport
  cmd_lateral_velocity_-1_1 : Inport  Port=2
  initial_horizontal_position : Inport  Port=3
  manual_mode : Inport  Port=4
  Bus Creator : BusCreator  Inputs=3
  Bus Selector2 : BusSelector  OutputSignals=x_ref,x_dt_ref
  Discrete-Time Integrator : DiscreteIntegrator  ExternalReset=rising  InitialConditionSource=external  SampleTime=-1  ICPrevOutput=DiscIntNeverNeededParam  ICPrevScaledInput=DiscIntNeverNeededParam
  Gain : Gain
  Gain1 : Gain
  Gain3 : Gain  Gain=horiz_pos_cntrl.rm.uv_max
  MATLAB Function1 : MATLAB Function  TreatAsAtomicUnit=on
  Mux : Mux  Inputs=2
  PT1 discrete reference model : ndi_lib/PT1 discrete reference model  T=horiz_pos_cntrl.rm.uv_T  x_max=inf  x_min=-inf  x_dt_max=horiz_pos_cntrl.rm.uv_dt_max  x_dt_min=-horiz_pos_cntrl.rm.uv_dt_max  x_init=0
      settings: SourceProductName=LADAC
  Product : Product
  Terminator : Terminator
  ny : Outport
  reference : Outport  Port=2
  wires:
  Gain3/1 -> Product/2
  Product/1 -> PT1 discrete reference model/1
  MATLAB Function1/1(cmd_velocity_abs_0_1) -> Gain3/1
  MATLAB Function1/2(lean_direction_angle) -> Terminator/1
  Mux/1 -> Product/1
  Gain1/1 -> Bus Creator/3, ny/1  "xy_g_dt2"
  Gain/1 -> Bus Creator/2  "xy_g_dt"
  cmd_lateral_velocity_-1_1/1 -> MATLAB Function1/1(stick_roll_cmd), Mux/2
  initial_horizontal_position/1 -> Discrete-Time Integrator/3
  Bus Selector2/2 -> Gain1/1  "<x_dt_ref>"
  Bus Selector2/1 -> Discrete-Time Integrator/1, Gain/1  "<x_ref>"
  Discrete-Time Integrator/1 -> Bus Creator/1  "xy_g"
  PT1 discrete reference model/1 -> Bus Selector2/1
  Bus Creator/1 -> reference/1
  cmd_forward_velocity_-1_1/1 -> MATLAB Function1/2(stick_pitch_cmd), Mux/1
  manual_mode/1 -> Discrete-Time Integrator/2

== system ArduCopter_MinnieTrajController/Multicopter INDI Loiter Flight Mode/Horizontal NDI position (NE) controller cascade with reduced attitude (angle) command/measures ==
  xy_g : Inport
  xy_g_dt : Inport  Port=2
  s_Kg_dt2 : Inport  Port=3
  Bus Creator1 : BusCreator  Inputs=4
  Selector3 : Selector  InputPortWidth=3  IndexOptions=Index vector (dialog)  Indices=[1,2]  OutputSizes=1
  Selector4 : Selector  InputPortWidth=3  IndexOptions=Index vector (dialog)  Indices=[1,2]  OutputSizes=1
  Selector5 : Selector  InputPortWidth=3  IndexOptions=Index vector (dialog)  Indices=[1,2]  OutputSizes=1
  Selector6 : Selector  InputPortWidth=3  IndexOptions=Index vector (dialog)  Indices=3  OutputSizes=1
  measure : Outport
  wires:
  s_Kg_dt2/1 -> Selector6/1, Selector5/1
  xy_g_dt/1 -> Selector4/1
  xy_g/1 -> Selector3/1
  Selector4/1 -> Bus Creator1/2  "xy_g_dt"
  Selector3/1 -> Bus Creator1/1  "xy_g"
  Selector5/1 -> Bus Creator1/3  "xy_g_dt2"
  Selector6/1 -> Bus Creator1/4  "z_g_dt2"
  Bus Creator1/1 -> measure/1

== system ArduCopter_MinnieTrajController/Multicopter INDI Loiter Flight Mode/Horizontal NDI position (NE) controller cascade with reduced attitude (angle) command/position controller ==
  reference : Inport
  measure : Inport  Port=2
  Add : Sum  Inputs=+-
  Bus Selector : BusSelector  OutputSignals=xy_g,xy_g_dt,xy_g_dt2
  Bus to Vector : BusToVector
  Gain : Gain  Gain=horiz_pos_cntrl.K  Multiplication=Matrix(K*u)
  Mux : Mux  Inputs=3
  PT2 discrete with saturation : filters_lib/PT2 discrete with saturation  omega=2./T  d=1  x_dt2_max=inf  x_dt2_min=-inf  x_dt_max=inf  x_dt_min=-inf  x_max=inf  x_min=-inf  x_init=0  x_dt_init=0
      settings: SourceProductName=LADAC
  Saturation : Saturate  UpperLimit=horiz_pos_cntrl.limits.uv_dt_max  LowerLimit=-horiz_pos_cntrl.limits.uv_dt_max
  Saturation1 : Saturate  UpperLimit=[horiz_pos_cntrl.limits.e_xy_max;1000;1000;1000;1000]  LowerLimit=-[horiz_pos_cntrl.limits.e_xy_max;1000;1000;1000;1000]
  Terminator : Terminator
  Terminator1 : Terminator
  ny_cntrl : Outport
  e : Outport  Port=2
  wires:
  PT2 discrete with saturation/1 -> Add/1
  PT2 discrete with saturation/3 -> Terminator1/1
  PT2 discrete with saturation/2 -> Terminator/1
  Bus to Vector/1 -> PT2 discrete with saturation/1
  Bus Selector/1 -> Mux/1  "<xy_g>"
  Bus Selector/2 -> Mux/2  "<xy_g_dt>"
  Bus Selector/3 -> Mux/3  "<xy_g_dt2>"
  Mux/1 -> Add/2
  measure/1 -> Bus Selector/1
  Gain/1 -> Saturation/1
  Saturation1/1 -> Gain/1
  Saturation/1 -> ny_cntrl/1
  Add/1 -> e/1, Saturation1/1
  reference/1 -> Bus to Vector/1

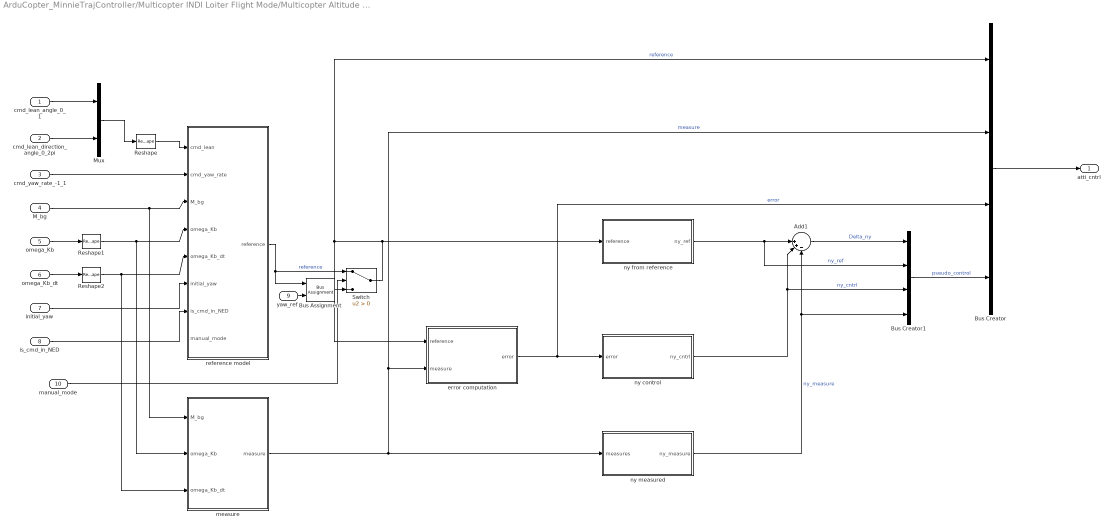
== system ArduCopter_MinnieTrajController/Multicopter INDI Loiter Flight Mode/Multicopter Altitude Hold Flight Mode with INDI and reduced attitude control/Multicopter (Reduced) Attitude INDI Controller ==
  cmd_lean_angle_0_1 : Inport
  cmd_lean_direction_angle_0_2pi : Inport  Port=2
  cmd_yaw_rate_-1_1 : Inport  Port=3
  M_bg : Inport  Port=4
  omega_Kb : Inport  Port=5
  omega_Kb_dt : Inport  Port=6
  initial_yaw : Inport  Port=7
  is_cmd_in_NED : Inport  Port=8
  "yaw_ref " : Inport  Port=9
  manual_mode : Inport  Port=10
  Add1 : Sum  Inputs=||++-
  Bus Assignment : BusAssignment  AssignedSignals=yaw
  Bus Creator : BusCreator  Inputs=4
  Bus Creator1 : BusCreator  Inputs=4
  Mux : Mux  Inputs=2
  Reshape : Reshape  OutputDimensionality=Column vector (2-D)
  Reshape1 : Reshape  OutputDimensionality=Column vector (2-D)
  Reshape2 : Reshape  OutputDimensionality=Column vector (2-D)
  Switch : Switch  Criteria=u2 > Threshold
  error computation : Subsystem
  measure : Subsystem
  ny control : Subsystem
  ny from reference : Subsystem
  ny measured : Subsystem
  reference model : Subsystem
  atti_cntrl : Outport
  wires:
  is_cmd_in_NED/1 -> reference model/7(is_cmd_in_NED)
  cmd_yaw_rate_-1_1/1 -> reference model/2(cmd_yaw_rate)
  cmd_lean_direction_angle_0_2pi/1 -> Mux/2
  cmd_lean_angle_0_1/1 -> Mux/1
  Reshape2/1 -> reference model/5(omega_Kb_dt), measure/3(omega_Kb_dt)
  Reshape1/1 -> reference model/4(omega_Kb), measure/2(omega_Kb)
  Reshape/1 -> reference model/1(cmd_lean)
  measure/1(measure) -> ny measured/1(measures), error computation/2(measure), Bus Creator/2  "measure"
  omega_Kb/1 -> Reshape1/1
  M_bg/1 -> reference model/3(M_bg), measure/1(M_bg)
  Add1/1 -> Bus Creator1/1  "Delta_ny"
  Bus Creator1/1 -> Bus Creator/4  "pseudo_control"
  Bus Creator/1 -> atti_cntrl/1
  initial_yaw/1 -> reference model/6(initial_yaw)
  Switch/1 -> error computation/1(reference), Bus Creator/1, ny from reference/1(reference)  "reference"
  ny measured/1(ny_measure) -> Add1/3, Bus Creator1/4  "ny_measure"
  ny control/1(ny_cntrl) -> Add1/2, Bus Creator1/3  "ny_cntrl"
  omega_Kb_dt/1 -> Reshape2/1
  error computation/1(error) -> Bus Creator/3, ny control/1(error)  "error"
  Mux/1 -> Reshape/1
  ny from reference/1(ny_ref) -> Add1/1, Bus Creator1/2  "ny_ref"
  manual_mode/1 -> Switch/2
  "yaw_ref "/1 -> Bus Assignment/2
  reference model/1(reference) -> Switch/1, Bus Assignment/1  "reference"
  Bus Assignment/1 -> Switch/3

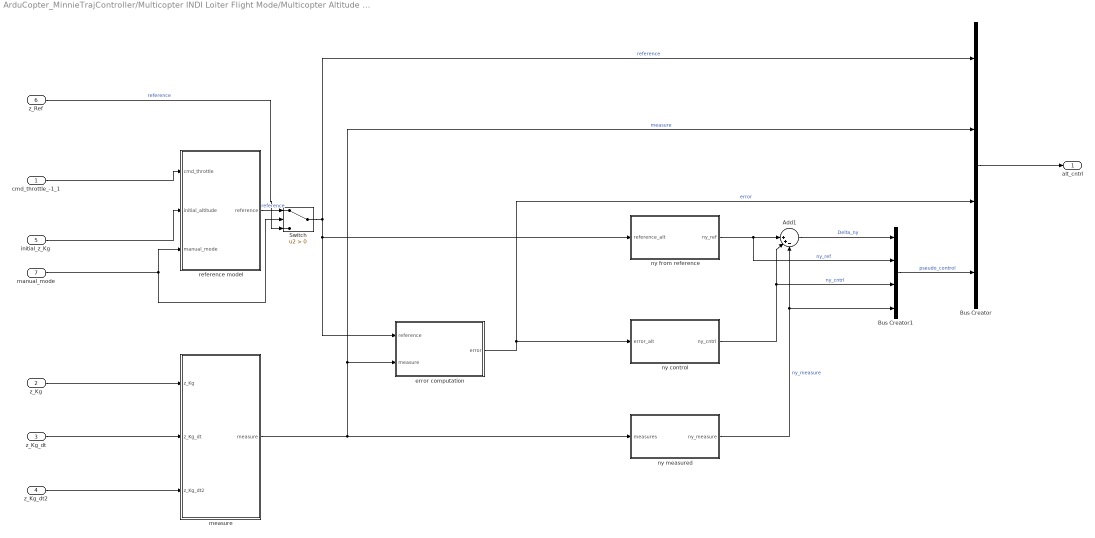
== system ArduCopter_MinnieTrajController/Multicopter INDI Loiter Flight Mode/Multicopter Altitude Hold Flight Mode with INDI and reduced attitude control/Multicopter Altitude INDI Controller1 ==
  cmd_throttle_-1_1 : Inport
  z_Kg : Inport  Port=2
  z_Kg_dt : Inport  Port=3
  z_Kg_dt2 : Inport  Port=4
  initial_z_Kg : Inport  Port=5
  z_Ref : Inport  Port=6
  manual_mode : Inport  Port=7
  Add1 : Sum  Inputs=||++-
  Bus Creator : BusCreator  Inputs=4
  Bus Creator1 : BusCreator  Inputs=4
  Switch : Switch  Criteria=u2 > Threshold
  error computation : Subsystem
  measure : Subsystem
  ny control : Subsystem
  ny from reference : Subsystem
  ny measured : Subsystem
  reference model : Subsystem
  alt_cntrl : Outport
  wires:
  cmd_throttle_-1_1/1 -> reference model/1(cmd_throttle)
  z_Kg/1 -> measure/1(z_Kg)
  z_Kg_dt/1 -> measure/2(z_Kg_dt)
  z_Kg_dt2/1 -> measure/3(z_Kg_dt2)
  measure/1(measure) -> error computation/2(measure), Bus Creator/2, ny measured/1(measures)  "measure"
  Add1/1 -> Bus Creator1/1  "Delta_ny"
  Bus Creator1/1 -> Bus Creator/4  "pseudo_control"
  Bus Creator/1 -> alt_cntrl/1
  initial_z_Kg/1 -> reference model/2(initial_altitude)
  Switch/1 -> Bus Creator/1, ny from reference/1(reference_alt), error computation/1(reference)  "reference"
  ny measured/1(ny_measure) -> Add1/3, Bus Creator1/4  "ny_measure"
  ny control/1(ny_cntrl) -> Add1/2, Bus Creator1/3  "ny_cntrl"
  error computation/1(error) -> Bus Creator/3, ny control/1(error_alt)  "error"
  ny from reference/1(ny_ref) -> Add1/1, Bus Creator1/2  "ny_ref"
  z_Ref/1 -> Switch/3  "reference"
  reference model/1(reference) -> Switch/1  "reference"
  manual_mode/1 -> Switch/2, reference model/3(manual_mode)

== system ArduCopter_MinnieTrajController/Multicopter INDI Loiter Flight Mode/Multicopter Altitude Hold Flight Mode with INDI and reduced attitude control/acceleration g to b frame ==
  z_Kg_dt2_cmd : Inport
  M_bg : Inport  Port=2
  MATLAB Function : MATLAB Function  TreatAsAtomicUnit=on
  dcm2Lean : MATLAB Function  TreatAsAtomicUnit=on
  z_Kb_dt2_cmd : Outport
  wires:
  dcm2Lean/1(phi) -> MATLAB Function/2(lean_angle)
  M_bg/1 -> dcm2Lean/1(M_bg)
  MATLAB Function/1(z_Kb_dt2_cmd) -> z_Kb_dt2_cmd/1
  z_Kg_dt2_cmd/1 -> MATLAB Function/1(z_Kg_dt2_cmd)

== system ArduCopter_MinnieTrajController/Multicopter INDI Loiter Flight Mode/Multicopter Altitude Hold Flight Mode with INDI and reduced attitude control/control effectiveness ==
  u : Inport
  Constant : Constant  Value=fm.cntrl_effect.u_trim  OutDataTypeStr=single
  Constant1 : Constant  Value=fm.ca.u_min  OutDataTypeStr=single
  Constant4 : Constant  Value=fm.sample_time  OutDataTypeStr=single
  MATLAB Function : MATLAB Function  TreatAsAtomicUnit=on
  Max : MinMax  Function=max  Inputs=2  OutDataTypeStr=Inherit: Inherit via back propagation
  ny_du_dt : Constant  Value=fm.cntrl_effect.ny_du_dt  OutDataTypeStr=single
  ny_du_red_trim : Constant  Value=fm.cntrl_effect.ny_du_red  OutDataTypeStr=single
  G1 : Outport
  G2 : Outport  Port=2
  wires:
  ny_du_red_trim/1 -> MATLAB Function/1(ny_du_red_trim)
  Constant4/1 -> MATLAB Function/5(T_s)
  Constant/1 -> MATLAB Function/3(u_trim)
  ny_du_dt/1 -> MATLAB Function/2(ny_du_dt_trim)
  u/1 -> Max/1
  Constant1/1 -> Max/2
  Max/1 -> MATLAB Function/4(u)
  MATLAB Function/1(G1) -> G1/1
  MATLAB Function/2(G2) -> G2/1

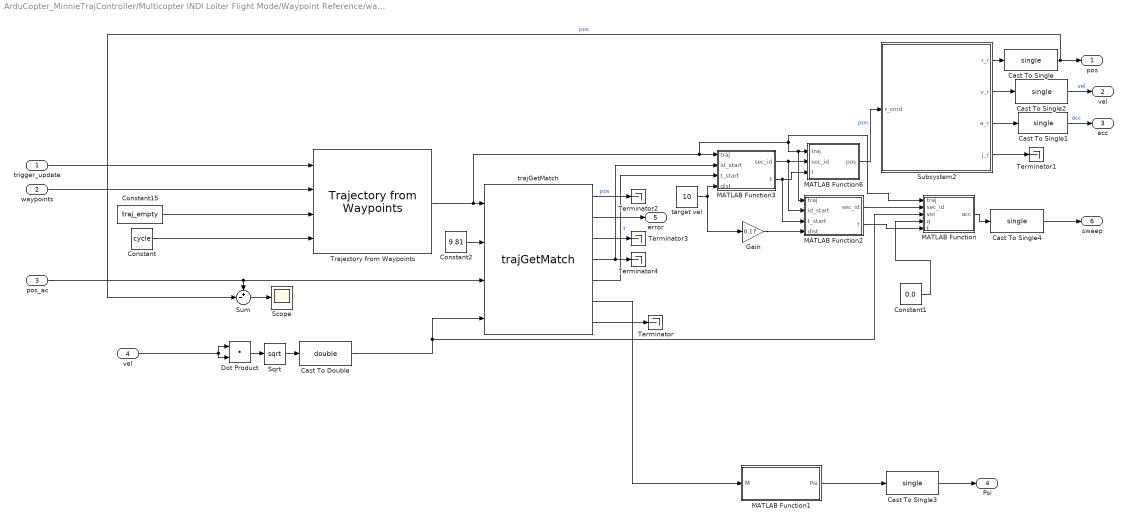
== system ArduCopter_MinnieTrajController/Multicopter INDI Loiter Flight Mode/Waypoint Reference/waypoint Reference System ==
  trigger_update : Inport
  waypoints : Inport  Port=2
  pos_ac : Inport  Port=3
  "vel " : Inport  Port=4
  Cast To Double : DataTypeConversion  OutDataTypeStr=double
  Cast To Single{,1..4} (5 alike) : DataTypeConversion  OutDataTypeStr=single
  Constant : Constant  Value=cycle
  Constant1 : Constant  Value=0.0
  Constant15 : Constant  Value=traj_empty  OutDataTypeStr=Bus: trajectoryBus
  Constant2 : Constant  Value=9.81
  Dot Product : DotProduct  InputSameDT=on  OutDataTypeStr=Inherit: Inherit via internal rule
  Gain : Gain  Gain=0.17
  MATLAB Function : MATLAB Function  TreatAsAtomicUnit=on
  MATLAB Function1 : MATLAB Function  TreatAsAtomicUnit=on
  MATLAB Function2 : MATLAB Function  TreatAsAtomicUnit=on
  MATLAB Function3 : MATLAB Function  TreatAsAtomicUnit=on
  MATLAB Function6 : MATLAB Function  TreatAsAtomicUnit=on
  Scope : Scope
  Sqrt : Sqrt  SaturateOnIntegerOverflow=on
  Subsystem2 : Subsystem
  Sum : Sum  Inputs=+-|
  Terminator{,1..4} (5 alike) : Terminator
  Trajectory from Waypoints : traj_lib/Trajectory from Waypoints
      settings: SourceProductName=LADAC
  target vel : Constant  Value=10
  trajGetMatch : traj_lib/trajGetMatch  SystemSampleTime=-1
      settings: SourceProductName=LADAC
  pos : Outport
  vel : Outport  Port=2
  acc : Outport  Port=3
  Psi : Outport  Port=4
  error : Outport  Port=5
  "sweep " : Outport  Port=6
  wires:
  Constant15/1 -> Trajectory from Waypoints/3
  waypoints/1 -> Trajectory from Waypoints/2
  trajGetMatch/4 -> MATLAB Function3/2(id_start), Terminator4/1
  "vel "/1 -> Dot Product/2, Dot Product/1
  Cast To Single1/1 -> acc/1  "acc"
  pos_ac/1 -> trajGetMatch/3, Sum/1
  Cast To Single2/1 -> vel/1  "vel"
  Cast To Single/1 -> Sum/2, pos/1  "pos"
  trajGetMatch/3 -> Terminator3/1
  Constant/1 -> Trajectory from Waypoints/4
  Constant2/1 -> trajGetMatch/2
  trajGetMatch/6 -> MATLAB Function1/1(M)
  trajGetMatch/5 -> MATLAB Function3/3(t_start)  "t"
  trigger_update/1 -> Trajectory from Waypoints/1
  trajGetMatch/2 -> error/1
  Cast To Single3/1 -> Psi/1
  MATLAB Function1/1(Psi) -> Cast To Single3/1
  Sum/1 -> Scope/1
  Dot Product/1 -> Sqrt/1
  Cast To Double/1 -> MATLAB Function/3(vel), trajGetMatch/4
  MATLAB Function3/1(sec_id) -> MATLAB Function2/2(id_start), MATLAB Function6/2(sec_id)
  Subsystem2/1(r_r) -> Cast To Single/1
  Subsystem2/2(v_r) -> Cast To Single2/1
  Subsystem2/3(a_r) -> Cast To Single1/1
  trajGetMatch/1 -> Terminator2/1  "pos"
  MATLAB Function6/1(pos) -> Subsystem2/1(r_cmd)  "pos"
  target vel/1 -> MATLAB Function3/4(dist), Gain/1
  Sqrt/1 -> Cast To Double/1
  trajGetMatch/7 -> Terminator/1
  Subsystem2/4(j_r) -> Terminator1/1
  MATLAB Function3/2(t) -> MATLAB Function2/3(t_start), MATLAB Function6/3(t)
  Gain/1 -> MATLAB Function2/4(dist)
  MATLAB Function2/2(t) -> MATLAB Function/5(t)
  MATLAB Function2/1(sec_id) -> MATLAB Function/2(sec_id)
  Constant1/1 -> MATLAB Function/4(g)
  MATLAB Function/1(acc) -> Cast To Single4/1
  Cast To Single4/1 -> "sweep "/1
  Trajectory from Waypoints/1 -> MATLAB Function/1(traj), MATLAB Function2/1(traj), MATLAB Function6/1(traj), MATLAB Function3/1(traj), trajGetMatch/1

== system ArduCopter_MinnieTrajController/Multicopter INDI Loiter Flight Mode/Delta attitude to stick commands/conversion to total attitude command/quaternion to lean angles ==
  q_bg : Inport
  MATLAB Function4 : MATLAB Function  TreatAsAtomicUnit=on
  quaternion to reduced attitude unit vector : MATLAB Function  TreatAsAtomicUnit=on
  phi : Outport
  delta : Outport  Port=2
  wires:
  MATLAB Function4/2(delta) -> delta/1
  q_bg/1 -> quaternion to reduced attitude unit vector/1(q_bg)
  MATLAB Function4/1(phi) -> phi/1
  quaternion to reduced attitude unit vector/1(n_g) -> MATLAB Function4/1(n_g)
